simulink model "scheme1"  (R2014a)
settings: Solver=ode45  StartTime=0.0  StopTime=5  MaxStep=0.001  MinStep=0.0001  RelTol=1e-3
settings Model: Creator=Valentin  LastModifiedBy=Valentin

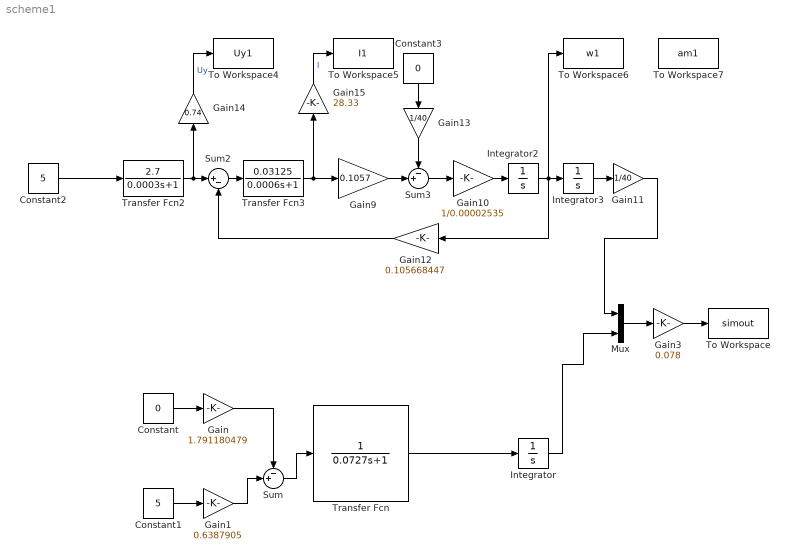
== system scheme1 ==
  Constant : Constant  Value=0
  Constant1 : Constant  Value=5
  Constant2 : Constant  Value=5
  Constant3 : Constant  Value=0
  Gain : Gain  Gain=1.791180479
  Gain1 : Gain  Gain=0.6387905
  Gain10 : Gain  Gain=1/0.00002535
  Gain11 : Gain  Gain=1/40
  Gain12 : Gain  Gain=0.105668447
  Gain13 : Gain  Gain=1/40
  Gain14 : Gain  Gain=0.74
  Gain15 : Gain  Gain=28.33
  Gain3 : Gain  Gain=0.078
  Gain9 : Gain  Gain=0.1057
  Integrator : Integrator
  Integrator2 : Integrator
  Integrator3 : Integrator
  Mux : Mux  Inputs=2
  Sum : Sum  Inputs=-+|
  Sum2 : Sum  Inputs=|+-
  Sum3 : Sum  Inputs=-+|
  To Workspace : ToWorkspace  VariableName=simout  SaveFormat=Timeseries  SampleTime=-1
  To Workspace4 : ToWorkspace  VariableName=Uy1  SaveFormat=Timeseries  SampleTime=-1
  To Workspace5 : ToWorkspace  VariableName=I1  SaveFormat=Timeseries  SampleTime=-1
  To Workspace6 : ToWorkspace  VariableName=w1  SaveFormat=Timeseries  SampleTime=-1
  To Workspace7 : ToWorkspace  VariableName=am1  SaveFormat=Timeseries  SampleTime=-1
  Transfer Fcn : TransferFcn  Denominator=[0.0727 1]
  Transfer Fcn2 : TransferFcn  Numerator=[2.7]  Denominator=[0.0003 1]
  Transfer Fcn3 : TransferFcn  Numerator=[0.03125]  Denominator=[0.0006 1]
  wires:
  Transfer Fcn2/1 -> Sum2/1, Gain14/1
  Sum2/1 -> Transfer Fcn3/1
  Transfer Fcn3/1 -> Gain15/1, Gain9/1
  Gain9/1 -> Sum3/2
  Gain13/1 -> Sum3/1
  Constant2/1 -> Transfer Fcn2/1
  Constant3/1 -> Gain13/1
  Sum3/1 -> Gain10/1
  Gain10/1 -> Integrator2/1
  Integrator2/1 -> To Workspace6/1, Integrator3/1, Gain12/1
  Integrator3/1 -> Gain11/1
  Gain12/1 -> Sum2/2
  Gain14/1 -> To Workspace4/1  "Uy"
  Gain15/1 -> To Workspace5/1  "I"
  Constant/1 -> Gain/1
  Constant1/1 -> Gain1/1
  Gain/1 -> Sum/1
  Gain1/1 -> Sum/2
  Sum/1 -> Transfer Fcn/1
  Transfer Fcn/1 -> Integrator/1
  Integrator/1 -> Mux/2
  Mux/1 -> Gain3/1
  Gain3/1 -> To Workspace/1
  Gain11/1 -> Mux/1
